simulink model "population_model"  (R2014b)
settings: Solver=ode45  StartTime=0.0  StopTime=500  RelTol=1e-3
settings Model: Creator=Shane Reynolds  LastModifiedBy=Shane Reynolds

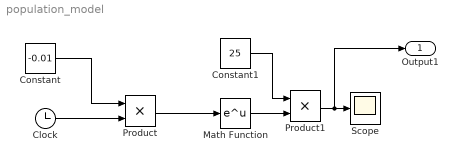
== system population_model ==
  Clock : Clock
  Constant : Constant  Value=-0.01
  Constant1 : Constant  Value=25
  Math Function : Math  SaturateOnIntegerOverflow=on
  Product : Product
  Product1 : Product
  Scope : Scope
  Output1 : Outport
  wires:
  Clock/1 -> Product/2
  Product/1 -> Math Function/1
  Constant/1 -> Product/1
  Math Function/1 -> Product1/2
  Constant1/1 -> Product1/1
  Product1/1 -> Output1/1, Scope/1
